simulink model "buckboost_CMC_compensator"  (R2024b)
settings: Solver=ode23s  StartTime=0.0  StopTime=0.03  FixedStep=1e-6  MaxStep=1e-7  RelTol=1e-7
values from neighbouring files (symbols this model uses):
  A = 80000    [Buck_boost_DCM.m]    (also in buckboost.m)
  C = 78.8e-6    (= 7.88e-05)    [Buck_boost_DCM.m]    (also in Input_Filter.m; buckboost.m)
  fs = 300e3    (= 300000)    [Buck_boost_DCM.m]    (also in Input_Filter.m; buckboost.m)
  L = 22e-6    (= 2.2e-05)    [Buck_boost_DCM.m]    (also in Input_Filter.m; buckboost.m)
  R4 = 1.13e3    (= 1130)    [Buck_boost_DCM.m]    (also in buckboost.m)
  R5 = 10e3    (= 10000)    [Buck_boost_DCM.m]    (also in buckboost.m)
  Ri = 0.3    [Buck_boost_DCM.m]    (also in Input_Filter.m; buckboost.m)
  Se = 90000    [Input_Filter.m]    (also in buckboost.m)
  Vdc = 24    [Buck_boost_DCM.m]    (also in Input_Filter.m; buckboost.m)
  Vref = 1.215    [Buck_boost_DCM.m]    (also in Input_Filter.m; buckboost.m)
  wpc = 14e4    (= 140000)    [buckboost.m]
  wzc = 5000    [buckboost.m]
undefined symbols (not defined in the file or in its folder): sigbuilder_block
libraries: spsSeriesRLCBranchLib x5, spsCurrentMeasurementLib x2, spsVoltageMeasurementLib x2, spsControlledCurrentSourceLib x1, spsDiodeLib x1, spsDCVoltageSourceLib x1, spsMosfetLib x1, simulink x1, spspowerguiLib x1
settings Model: Creator=Fahd Fakhry  LastModifiedBy=moham
settings SolverCC: ZeroCrossAlgorithm=Adaptive
settings DebuggingCC: IgnoredZcDiagnostic=none  UnconnectedInputMsg=warning  UnconnectedOutputMsg=warning  UnconnectedLineMsg=warning
settings ModelReferenceCC: EnableRefExpFcnMdlSchedulingChecks=on
settings RTWCC: GPUComputeCapability=3.5  DLArmComputeVersion=19.05

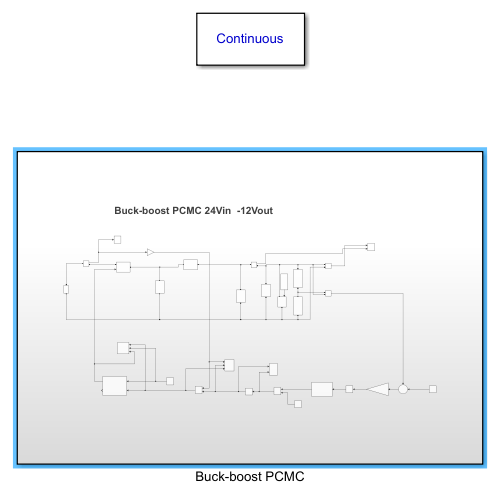
[thumbnail: Simulink's stored preview of the top-level diagram]
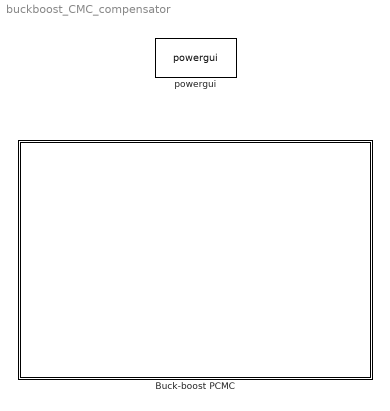
== system buckboost_CMC_compensator ==
  Buck-boost PCMC : Subsystem
  powergui : spspowerguiLib/powergui  Priority=1  SimulationMode=Continuous  SampleTime=50e-6  frequency=60  Iterations=50  frequencyindice=0  Pbase=100e6  ErrMax=1e-4  UnitsV=kV  UnitsW=MW  buscounter=0  FunctionMessages=off  echomessages=off  EnableUseOfTLC=off  CurrentSourceSwitches=off  DisableSnubberDevices=off  DisableRonSwitches=off  DisableVfSwitches=off  DisplayEquations=off  AutomaticDiscreteSolvers=off  SolverType=Tustin/Backward Euler (TBE)  Interpol=off  ExternalGateDelay=off  methode=off  Ts=100  x0status=blocks  SPID=on  SwTol=0  HookPort=off  NonlinearTolerance=1e-4  nMaxIteration=100  ContinueOnMaxIteration=off  RestoreLinks=warning  ResistiveCurrentMeasurement=off  Frange=[0:2:500]  Ylog=off  Xlog=on  ShowGrid=off  save=off  variable=ZData  structure=0  ZoomFFT=off  StartTime=0.0  cycles=1  DisplayStyle=1  fundamental=60  FreqAxis=off  MaxFrequency=1000  frequencyindicesteady=1  RmsSteady=1  display=off

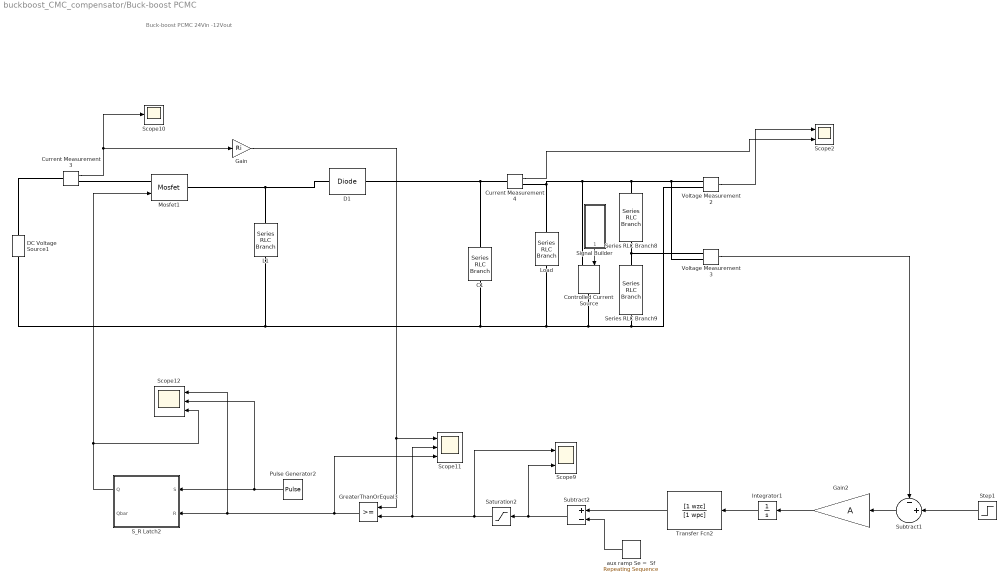
== system buckboost_CMC_compensator/Buck-boost PCMC ==
  note: Buck-boost PCMC 24Vin -12Vout
  C1 : spsSeriesRLCBranchLib/Series RLC Branch  LConnTagsString=__new0  RConnTagsString=__new0  BranchType=C  Resistance=1  Inductance=1e-3  SetiL0=off  InitialCurrent=0  Capacitance=C  Setx0=off  InitialVoltage=0  Measurements=None
  Controlled Current Source : spsControlledCurrentSourceLib/Controlled Current Source  Initialize=on  Source_Type=DC  Amplitude=0  Phase=0  Frequency=0  Measurements=None
  Current Measurement3 : spsCurrentMeasurementLib/Current Measurement  PhasorSimulation=off  OutputType=Complex  PSBequivalent=0
  Current Measurement4 : spsCurrentMeasurementLib/Current Measurement  PhasorSimulation=off  OutputType=Complex  PSBequivalent=0
  D1 : spsDiodeLib/Diode  Ron=0.001  Lon=0  Vf=0.8  IC=0  UseSnubber=0  Rs=500  Cs=250e-9  Measurements=off
  DC Voltage Source1 : spsDCVoltageSourceLib/DC Voltage Source  Amplitude=Vdc  Measurements=None
  Gain : Gain  Gain=Ri
  Gain2 : Gain  Gain=A
  GreaterThanOrEqual3 : RelationalOperator  OutDataTypeStr=boolean  RndMeth=Simplest  InputSameDT=off
  Integrator1 : Integrator
  L1 : spsSeriesRLCBranchLib/Series RLC Branch  LConnTagsString=__new0  RConnTagsString=__new0  BranchType=L  Resistance=1  Inductance=L  SetiL0=off  InitialCurrent=0  Capacitance=1e-6  Setx0=off  InitialVoltage=0  Measurements=None
  Load : spsSeriesRLCBranchLib/Series RLC Branch  LConnTagsString=__new0  RConnTagsString=__new0  BranchType=R  Resistance=10  Inductance=1e-3  SetiL0=off  InitialCurrent=0  Capacitance=1e-6  Setx0=off  InitialVoltage=0  Measurements=None
  Mosfet1 : spsMosfetLib/Mosfet  Ron=0.01  Lon=0  Rd=0.02  Vfd=0  IC=0  Rs=1e5  Cs=inf  Measurements=off
  Pulse Generator2 : DiscretePulseGenerator  PulseType=Time based  Period=3.333e-6
  S_R Latch2 : MATLAB Function  TreatAsAtomicUnit=on
  Saturation2 : Saturate  UpperLimit=15*Ri  LowerLimit=0.2
  Scope10 : Scope
  Scope11 : Scope  NumInputPorts=3
  Scope12 : Scope  NumInputPorts=3
  Scope2 : Scope  NumInputPorts=2
  Scope9 : Scope  NumInputPorts=2
  Series RLC Branch8 : spsSeriesRLCBranchLib/Series RLC Branch  LConnTagsString=__new0  RConnTagsString=__new0  BranchType=R  Resistance=R4  Inductance=220e-6  SetiL0=off  InitialCurrent=0  Capacitance=10e-6  Setx0=off  InitialVoltage=0  Measurements=None
  Series RLC Branch9 : spsSeriesRLCBranchLib/Series RLC Branch  LConnTagsString=__new0  RConnTagsString=__new0  BranchType=R  Resistance=R5  Inductance=220e-6  SetiL0=off  InitialCurrent=0  Capacitance=10e-6  Setx0=off  InitialVoltage=0  Measurements=None
  Signal Builder : Subsystem  Tag=STV Subsys  LoadFcn=sigbuilder_block('load');  StartFcn=sigbuilder_block('start');  StopFcn=sigbuilder_block('stop');  ClipboardFcn=sigbuilder_block('clipboard');  mask(Sigbuilder block){tuvar=[0:10]}
      mask help: Simulink:masks:SigbuilderBlock_MD
      mask init:
      | if ~strcmp(get_param(bdroot(gcbh),'SimulationStatus'),'stopped') tuvar = sigbuilder_block('maskInit'); end
      settings: CopyFcn=sigbuilder_block('copy');  DeleteFcn=sigbuilder_block('delete');  ModelCloseFcn=sigbuilder_block('modelClose');  PreSaveFcn=sigbuilder_block('preSave');  PauseFcn=sigbuilder_block('pause');  ContinueFcn=sigbuilder_block('continue');  NameChangeFcn=sigbuilder_block('namechange');  OpenFcn=sigbuilder_block('open',[5.4 36 1141.2 516.6 ]);  CloseFcn=sigbuilder_block('close');
      mask Display: plot(0, 0, 100, 100,[2, 2, 32, 32, 2], [68, 8, 8, 68, 68],[32, 2], [38, 38], [32, 19, 2],[53, 60, 44], [32, 17, 17, 2],[16, 16, 31, 31]);txt = getActiveGroup(gcbh);text(2, 100, txt,'verticalAlignment', 'top');
  Step1 : Step  Time=0.015  Before=Vref  After=Vref  SampleTime=0
  Subtract1 : Sum  Inputs=-+|
  Subtract2 : Sum  Inputs=+-
  Transfer Fcn2 : TransferFcn  Numerator=[1 wzc]  Denominator=[1 wpc]
  Voltage Measurement2 : spsVoltageMeasurementLib/Voltage Measurement  PhasorSimulation=off  OutputType=Complex  PSBequivalent=0
  Voltage Measurement3 : spsVoltageMeasurementLib/Voltage Measurement  PhasorSimulation=off  OutputType=Complex  PSBequivalent=0
  aux ramp Se =  Sf : simulink/Sources/Repeating Sequence  rep_seq_t=[0 (1/fs)]  rep_seq_y=[0 Se*(1/fs)*Ri]
  wires:
  Transfer Fcn2/1 -> Subtract2/1
  Pulse Generator2/1 -> Scope12/2, S_R Latch2/1(S)
  GreaterThanOrEqual3/1 -> S_R Latch2/2(R), Scope12/1, Scope11/3
  S_R Latch2/1(Q) -> Mosfet1/1, Scope12/3
  Subtract2/1 -> Saturation2/1, Scope9/2
  Current Measurement4/1 -> Scope2/2
  Subtract1/1 -> Gain2/1
  Step1/1 -> Subtract1/2
  Gain2/1 -> Integrator1/1
  Integrator1/1 -> Transfer Fcn2/1
  Voltage Measurement3/1 -> Subtract1/1
  Voltage Measurement2/1 -> Scope2/1
  Current Measurement3/1 -> Gain/1, Scope10/1
  Gain/1 -> GreaterThanOrEqual3/1, Scope11/1
  Saturation2/1 -> Scope9/1, GreaterThanOrEqual3/2, Scope11/2
  Signal Builder/1(Signal 1) -> Controlled Current Source/1
  aux ramp Se =  Sf/1 -> Subtract2/2
  connections:
  Controlled Current Source/LConn1 -- Voltage Measurement3/LConn2 -- Voltage Measurement2/LConn1 -- Series RLC Branch8/LConn1 -- Load/RConn1 -- Current Measurement4/RConn1
  Mosfet1/RConn1 -- D1/RConn1 -- L1/LConn1
  C1/LConn1 -- Load/LConn1 -- Controlled Current Source/RConn1 -- Voltage Measurement2/LConn2 -- Series RLC Branch9/RConn1 -- L1/RConn1 -- DC Voltage Source1/LConn1
  Series RLC Branch9/LConn1 -- Voltage Measurement3/LConn1 -- Series RLC Branch8/RConn1
  Current Measurement4/LConn1 -- C1/RConn1 -- D1/LConn1
  Mosfet1/LConn1 -- Current Measurement3/RConn1
  Current Measurement3/LConn1 -- DC Voltage Source1/RConn1

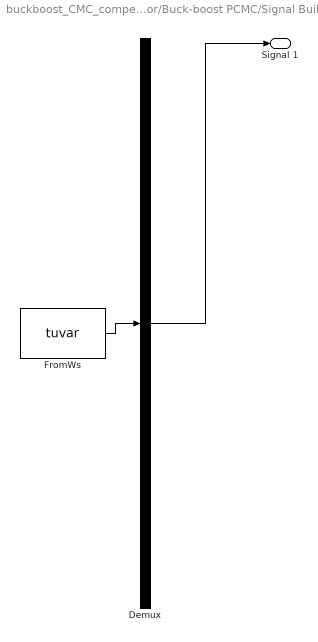
== system buckboost_CMC_compensator/Buck-boost PCMC/Signal Builder ==
  Demux : Demux  Tag=STV Demux  Outputs=1
      settings: DisplayOption=none
  FromWs : FromWorkspace  Tag=STV FromWs  VariableName=tuvar
      SigBuilderData=|
      | common.afterFinalStr = 'Extrapolate'
      | common.sampleTime = 0
      | dataSet.timeRange = [0 0.03]
      | dataSet.name = 'Group 1'
      | sbobj.Groups.Name = 'Group 1'
      | sbobj.Groups.Signals.Name = 'Signal 1'
      | sbobj.Groups.Signals.XData = [0 0.015 0.015 0.02 0.02 0.03]
      | sbobj.Groups.Signals.YData = [0 0 0.5 0.5 0 0]
      | sbobj.Groups.TimeRange = [0 0.03]
  Signal 1 : Outport  Tag=STV Outport
  wires:
  Demux/1 -> Signal 1/1
  FromWs/1 -> Demux/1

== matlab function buckboost_CMC_compensator/Buck-boost PCMC/S_R Latch2 ==
  data: S input; Q output; R input; Qbar output
function [Q, Qbar] = SR_latch(S, R)
    persistent Q_prev Qbar_prev;
    if isempty(Q_prev)
        Q_prev = 0;
        Qbar_prev = 1;
    end
    
    % Set Q and Qbar based on inputs S and R
    if S == 1 && R == 0
        Q = 1;
        Qbar = 0;
    elseif S == 0 && R == 1
        Q = 0;
        Qbar = 1;
    elseif S == 0 && R == 0
        Q = Q_prev;
        Qbar = Qbar_prev;
    elseif S == 1 && R == 1
        Q = 0; % Modified behavior: If both S and R are 1, Q is set to 0
        Qbar = 1;
    else
        % Invalid input combination
        error('Invalid input combination: S = %d, R = %d', S, R);
    end
    
    % Update previous values for next iteration
    Q_prev = Q;
    Qbar_prev = Qbar;
end
